simulink model "trans"  (R2013a)
settings: Solver=ode45  StartTime=0.0  StopTime=10.0  RelTol=1e-3
values from neighbouring files (symbols this model uses):
  Cv1 = cp*gp*V1    (= 90000)    [skrypt.m]
  Cv2 = cp*gp*V2    (= 144000)    [skrypt.m]
  czas_skoku = 300    [skrypt.m]
  dTkz = 0    [skrypt.m]
  dTzew = 0    [skrypt.m]
  K0 = (cp*gp*fkN*0.7*(TkzN - T1N)) / (T1N - T2N)    (= 653.333333333)    [skrypt.m]
  K1 = (cp*gp*fkN*0.3*(TkzN-T1N)) / (T1N - TzewN)    (= 35)    [skrypt.m]
  K2 = ((cp*gp*fkN + K0)*(T1N-T2N)) / (T2N - TzewN)    (= 160)    [skrypt.m]
  T10 = (cp*gp*fk*Tkz + K1*Tzew + ((K0*K2*Tzew)/(K0+K2+cp*gp*fk))) / (cp*gp*fk + K1 + K0 - ((K0*(K0+cp*gp*fk))/(K0+K2+cp*gp*fk)))    [skrypt.m]
  T20 = ((K0+cp*gp*fk)*T10 + K2*Tzew) / (K0 + cp*gp*fk + K2)    [skrypt.m]
  Tkz = TkzN    (= 30)    [skrypt.m]
  Tzew = TzewN+i*5    [skrypt.m]
  w = cp*gp*fk    (= 233.333333333)    [skrypt.m]
settings Model: Creator=LAB320-1552  LastModifiedBy=Dawidek

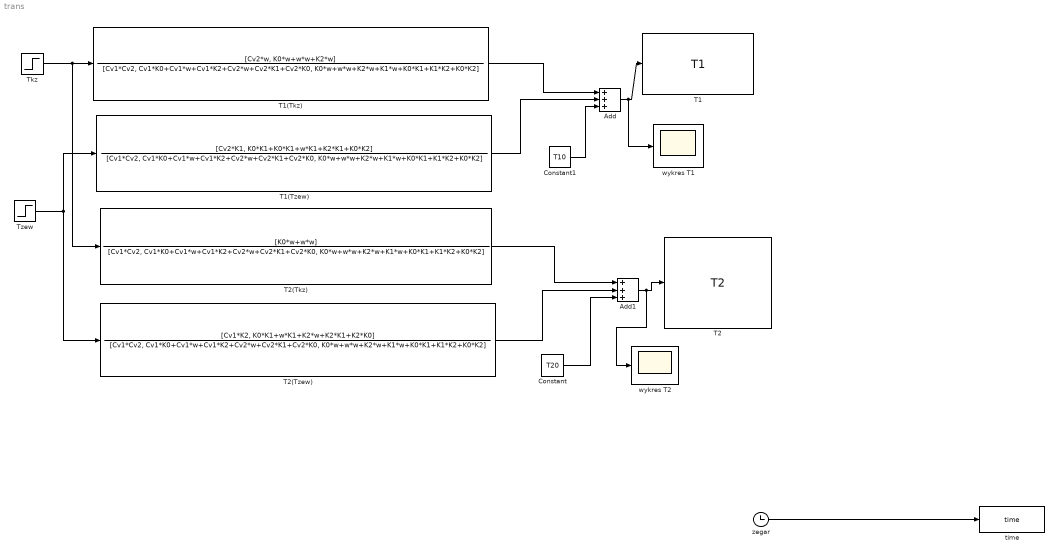
== system trans ==
  Add : Sum  Inputs=+++
  Add1 : Sum  Inputs=+++
  Constant : Constant  Value=T20
  Constant1 : Constant  Value=T10
  T1 : ToWorkspace  VariableName=T1  SampleTime=-1
  T1(Tkz) : TransferFcn  Numerator=[Cv2*w, K0*w+w*w+K2*w]  Denominator=[Cv1*Cv2, Cv1*K0+Cv1*w+Cv1*K2+Cv2*w+Cv2*K1+Cv2*K0, K0*w+w*w+K2*w+K1*w+K0*K1+K1*K2+K0*K2]
  T1(Tzew) : TransferFcn  Numerator=[Cv2*K1, K0*K1+K0*K1+w*K1+K2*K1+K0*K2]  Denominator=[Cv1*Cv2, Cv1*K0+Cv1*w+Cv1*K2+Cv2*w+Cv2*K1+Cv2*K0, K0*w+w*w+K2*w+K1*w+K0*K1+K1*K2+K0*K2]
  T2 : ToWorkspace  VariableName=T2  SampleTime=-1
  T2(Tkz) : TransferFcn  Numerator=[K0*w+w*w]  Denominator=[Cv1*Cv2, Cv1*K0+Cv1*w+Cv1*K2+Cv2*w+Cv2*K1+Cv2*K0, K0*w+w*w+K2*w+K1*w+K0*K1+K1*K2+K0*K2]
  T2(Tzew) : TransferFcn  Numerator=[Cv1*K2, K0*K1+w*K1+K2*w+K2*K1+K2*K0]  Denominator=[Cv1*Cv2, Cv1*K0+Cv1*w+Cv1*K2+Cv2*w+Cv2*K1+Cv2*K0, K0*w+w*w+K2*w+K1*w+K0*K1+K1*K2+K0*K2]
  Tkz : Step  Time=czas_skoku  After=Tkz+dTkz  SampleTime=0
  Tzew : Step  Time=czas_skoku  After=Tzew+dTzew  SampleTime=0
  time : ToWorkspace  VariableName=time  SampleTime=-1
  wykres T1 : Scope
      settings: TimeRange=10  YMin=-0.05  YMax=0
  wykres T2 : Scope
  zegar : Clock
  wires:
  zegar/1 -> time/1
  Tkz/1 -> T2(Tkz)/1, T1(Tkz)/1
  Tzew/1 -> T1(Tzew)/1, T2(Tzew)/1
  Add/1 -> wykres T1/1, T1/1
  Add1/1 -> wykres T2/1, T2/1
  Constant1/1 -> Add/3
  T1(Tzew)/1 -> Add/2
  T1(Tkz)/1 -> Add/1
  Constant/1 -> Add1/3
  T2(Tzew)/1 -> Add1/2
  T2(Tkz)/1 -> Add1/1
